simulink model "Simulacion_stepper"  (R2025b)
settings: Solver=ode4  StartTime=0.0  StopTime=Time_simulation  FixedStep=1/frecuency_simulation  RelTol=1e-3
InitFcn:
  | %%InitFcn();
StopFcn:
  | %%FinishFcn
model workspace (MAT data in the model file):
  Ts_stepper = 0.001
values from neighbouring files (symbols this model uses):
  B = motor_params.B_internal    [bode.m]    (also in current_observer.m = 0.0005; discretizacion.m = [ 1/L, 0; ekf_4_estados.m = params.B; obs_ctrl_back_emf_ext.m = [1/L 0)
  frecuency_simulation = 10e3    (= 10000)    [InitFcn.m]
  J = motor_params.J_internal    [bode.m]    (also in current_observer.m = 0.008; ekf_4_estados.m = params.J; obs_ctrl_back_emf_ext.m = 0.008; obs_y_contrl_back_emd.m = 0.008)
  Ke = 0.0055    [current_observer.m]    (also in ekf_4_estados.m = params.Ke; observer.m = Pvec(3); salient_motor.m = 0.0066)
  Ki_d = PI_dq_params.Ki_d_salient    [bode.m]
  Ki_q = PI_dq_params.Ki_q_salient    [bode.m]
  Ki_w = (wn_w^2)*J_var/Kt    [Barrido_B.m]    (also in Barrido_J.m; bode.m = PI_MTPA_params.Ki_w)
  Kp_d = PI_dq_params.Kp_d_salient    [bode.m]
  Kp_q = PI_dq_params.Kp_q_salient    [bode.m]
  Kp_w = (2*shi_w*wn_w*J_var)/Kt    [Barrido_B.m]    (also in Barrido_J.m; bode.m = PI_MTPA_params.Kp_w)
  Kt = Nr*Ke    (= 0.275)    [current_observer.m]    (also in ekf_4_estados.m = params.Kt; frecuencia_max.m = 0.33; observer.m = Pvec(4); salient_motor.m = 0.33)
  L = place(A', C', 10*eig(A)).'    [current_observer.m]    (also in desfase.m = lags(k); discretizacion.m = 0.01; frecuencia_max.m = 0.006; obs_ctrl_back_emf_ext.m = 0.006)
  P = motor_params.P    [bode.m]    (also in ekf_4_estados.m = P_pred; frecuencia_max.m = 50; salient_motor.m = 50)
  R = motor_params.R    [bode.m]    (also in current_observer.m = 3.4; discretizacion.m = 3.4; ekf_4_estados.m = params.R; frecuencia_max.m = 3.4)
  sample_time = 1/frecuency_simulation    (= 0.0001)    [InitFcn.m]
  Ts_current = 1/f_current    (= 0.0001)    [InitFcn.m]
  Ts_Wm = Ts_current*10    (= 0.001)    [InitFcn.m]
  Vdc = 24    [InitFcn.m]    (also in frecuencia_max.m = 12)
undefined symbols (not defined in the file or in its folder): DiscIntNeverNeededParam, EKF_params, motor_params, RI_base
libraries: simulink x8, mcbeeMathTransformLib x3, spspowerguiLib x1
(part 3 of 5)

== matlab function Simulacion_stepper/Motor 2 PI Speed MTPA2/MATLAB Function ==
  data: Wm_ref input; Wm input; Ts input; Kp_w input; Ki_w input; Kd_w input; Tf_w input; Tl_tdm input; B input; Imax input; RI_enable input; a_ri input; b_ri input; c_ri input; d_ri input; Kr_norm input; Ld input; Iq_ref output; Id_ref output; Iq_cogging output; Iq_PI output; Lq input; Ke input; P input; error_Wm output
function [Iq_ref, Id_ref, Iq_cogging, Iq_PI, error_Wm] = PI_speed_RI_MTPA( ...
        Wm_ref, Wm, Ts, ...
        Kp_w, Ki_w, Kd_w, Tf_w, ...
        Tl_tdm, B, ...
        Imax, ...
        RI_enable, a_ri, b_ri, c_ri, d_ri, Kr_norm, ...
        Ld, Lq, Ke, P)

% =========================================================================
% CONTROL DE VELOCIDAD Wm
%
% Incluye:
% - PI de velocidad.
% - Derivada opcional filtrada sobre la velocidad medida.
% - Compensación feedforward de carga/fricción.
% - Resonador opcional para cogging.
% - MTPA continuo.
% - Saturación vectorial de corriente.
% - Anti-windup del integrador de velocidad.
%
% Para usar solo PI:
%     Kd_w = 0;
%     RI_enable = 0;
% =========================================================================

% =========================================================================
% Estados persistentes
% =========================================================================
persistent int_w
persistent Wm_prev dWm_filt_prev
persistent y1_ri y2_ri
persistent e1_ri e2_ri

if isempty(int_w)

    int_w          = 0;

    Wm_prev        = 0;
    dWm_filt_prev  = 0;

    y1_ri          = 0;
    y2_ri          = 0;
    e1_ri          = 0;
    e2_ri          = 0;

end

% Protección numérica
Ts_eff   = max(Ts, 1e-9);
Imax_eff = max(abs(Imax), 1e-6);

% Constante de torque de reluctancia
Krel = P * (Lq - Ld);

% =========================================================================
% 1. Error de velocidad
% =========================================================================
error_Wm = Wm_ref - Wm;

% =========================================================================
% 2. Derivada filtrada sobre la velocidad medida
%
% Se usa derivada de Wm, no de error, para evitar golpes derivativos
% cuando cambia Wm_ref.
% =========================================================================
dWm_raw = (Wm - Wm_prev) / Ts_eff;

if Tf_w > 0
    alpha_d = Ts_eff / (Tf_w + Ts_eff);
    dWm_filt = dWm_filt_prev + alpha_d * (dWm_raw - dWm_filt_prev);
else
    dWm_filt = dWm_raw;
end

% Acción derivativa amortiguadora
D_w = -Kd_w * dWm_filt;

% =========================================================================
% 3. Feedforward de torque de carga y fricción
% =========================================================================
T_ff = Tl_tdm + B * Wm_ref;

if abs(Ke) > 1e-9
    Iq_ff = T_ff / Ke;
else
    Iq_ff = 0;
end

% =========================================================================
% 4. Resonador para compensación de ripple/cogging
% =========================================================================
if RI_enable == 1

    Iq_RI_new = ...
          c_ri * y1_ri ...
        - d_ri * y2_ri ...
        + Kr_norm * (error_Wm - a_ri * e1_ri + b_ri * e2_ri);

else
    Iq_RI_new = 0;
end

% =========================================================================
% 5. Integrador candidato
% =========================================================================
int_w_candidate = int_w + Ki_w * Ts_eff * error_Wm;

% =========================================================================
% 6. Cálculo PI/PID, MTPA y límite de corriente
%
% Se hacen hasta dos pasadas:
% - Primera: prueba integrando.
% - Segunda: si saturó y el integrador empeora la saturación,
%   se rechaza esa integración.
% =========================================================================
for pass = 1:2

    % Salida del controlador de velocidad
    Iq_PI = Kp_w * error_Wm + int_w_candidate + D_w;

    % Corriente q total solicitada
    Iq_ref_raw = Iq_ff + Iq_PI + Iq_RI_new;

    % =====================================================================
    % MTPA continuo
    %
    % Id_ref tiende suavemente a cero cuando Iq_ref_raw tiende a cero.
    % No existe umbral que fuerce saltos Id_ref = 0.
    % =====================================================================
    if abs(Krel) > 1e-9 && abs(Ke) > 1e-9

        A_mtpa = Ke / (2 * Krel);

        if abs(A_mtpa) > 1e-12

            % Forma numéricamente estable de:
            % Id = A - sign(A)*sqrt(A^2 + Iq^2)
            Id_ref_raw = -sign(A_mtpa) * (Iq_ref_raw^2) / ...
                (abs(A_mtpa) + sqrt(A_mtpa^2 + Iq_ref_raw^2));

        else
            Id_ref_raw = 0;
        end

    else
        Id_ref_raw = 0;
    end

    % =====================================================================
    % Saturación vectorial de corriente
    % =====================================================================
    Is_mag = sqrt(Id_ref_raw^2 + Iq_ref_raw^2);

    if Is_mag > Imax_eff

        ratio  = Imax_eff / Is_mag;

        Id_ref = Id_ref_raw * ratio;
        Iq_ref = Iq_ref_raw * ratio;

        sat = true;

    else

        Id_ref = Id_ref_raw;
        Iq_ref = Iq_ref_raw;

        sat = false;
    end

    % =====================================================================
    % Anti-windup condicional
    %
    % Si la salida está saturada y el error pide aumentar todavía más
    % la corriente saturada, no se integra.
    % Si el error ayuda a salir de saturación, sí se permite integrar.
    % =====================================================================
    integrator_worsens_sat = (Iq_ref_raw * error_Wm) >= 0;

    if pass == 1 && sat && integrator_worsens_sat

        % Rechaza la nueva integración y recalcula la salida.
        int_w_candidate = int_w;

    else
        break;
    end

end

% Guarda el integrador final
int_w = int_w_candidate;

% =========================================================================
% 7. Actualización de memorias
%
% Estas memorias se actualizan siempre, incluso durante saturación.
% =========================================================================
Wm_prev       = Wm;
dWm_filt_prev = dWm_filt;

if RI_enable == 1

    y2_ri = y1_ri;
    y1_ri = Iq_RI_new;

    e2_ri = e1_ri;
    e1_ri = error_Wm;

else

    % Evita que el resonador conserve memoria al desactivarlo.
    y1_ri = 0;
    y2_ri = 0;
    e1_ri = 0;
    e2_ri = 0;

end

% =========================================================================
% 8. Salidas de monitoreo
% =========================================================================
Iq_cogging = Iq_RI_new;

end

== matlab function Simulacion_stepper/Subsystem1/Triggered Subsystem4/MATLAB Function ==
  data: Wm_ref input; Wm input; Vd output; Vq output; Id output; Iq output; Iq_ref output; X input; Theta_e input; Ts input; Vdc input; Imax input; Kp_w input; Ki_w input; Kp_d input; Ki_d input; Kp_q input; Ki_q input; Tl_tdm input; B input; Kt input; Ke input; L input; P input; R input
function [Vd,Vq,Id,Iq,Iq_ref] = PI_dq( ...
        Wm_ref, Wm, X, Theta_e, Ts, Vdc, Imax, ...
        Kp_w, Ki_w, Kp_d, Ki_d, Kp_q, Ki_q, ...
        Tl_tdm, B, Kt, Ke, L, P,R)

% ===== FIX DIMENSIONES: preasignar salidas (escalares) =====
Vd     = 0.0;
Vq     = 0.0;
Id     = 0.0;
Iq     = 0.0;
Iq_ref = 0.0;

persistent ek_w ek1_w u_w ...
           ek_d ek1_d u_d ...
           ek_q ek1_q u_q

    if isempty(ek_w)
        ek_w  = 0;   ek1_w = 0;   u_w  = 0;
        ek_d  = 0;   ek1_d = 0;   u_d  = 0;
        ek_q  = 0;   ek1_q = 0;   u_q  = 0;
       
    end

    %% ================== Transformada dq ==================
    Ia = X(1);
    Ib = X(2);

    C = cos(Theta_e);
    S = sin(Theta_e);

    Id =  Ia*C + Ib*S;
    Iq = -Ia*S + Ib*C;   % signo correcto

    %% ================== Control de velocidad ==================
    ek1_w = ek_w;
    ek_w  = Wm_ref - Wm;

    k1_w = Kp_w + Ki_w*Ts;
    k2_w = -Kp_w;

    du_w = k1_w*ek_w + k2_w*ek1_w;
    u_w  = u_w + du_w;

    % Feedforward de torque
    Iq_ff  = (Tl_tdm + B*Wm)/Kt;
    Iq_ref = Iq_ff + u_w;

    % Saturación de corriente (Iq_ref ≤ Imax)
    if abs(Iq_ref) > Imax
        Iq_ref = sign(Iq_ref)*Imax;
        % anti-windup del PI de velocidad
        u_w  = u_w - du_w;
        ek_w = ek1_w;
    end

    %% ================== Control PI de Iq ==================
    ek1_q = ek_q;
    ek_q  = Iq_ref - Iq;

    k1_q = Kp_q + Ki_q*Ts;
    k2_q = -Kp_q;

    du_q = k1_q*ek_q + k2_q*ek1_q;
    u_q  = u_q + du_q;

    %% ================== Control PI de Id (Id_ref = 0) ==================
    ek1_d = ek_d;
    ek_d  = -Id;

    k1_d = Kp_d + Ki_d*Ts;
    k2_d = -Kp_d;

    du_d = k1_d*ek_d + k2_d*ek1_d;
    u_d  = u_d + du_d;

    %% ================== DESACOPLES ==================
    We = P * Wm;   % velocidad eléctrica

    Vdec_d = Id*R -L * We * Iq;
    Vdec_q = Iq*R + Ke * Wm + L * We * Id;

    % Voltajes no saturados
    Vd = u_d + Vdec_d;
    Vq = u_q + Vdec_q;

    %% ================== SATURACIÓN CIRCULAR dq ==================
    Vnorm = sqrt(Vd^2 + Vq^2);

    if Vnorm > Vdc
        scale = Vdc / Vnorm;
        Vd_sat = Vd * scale;
        Vq_sat = Vq * scale;

        % Anti-windup PI de corriente
        u_d = Vd_sat - Vdec_d;
        u_q = Vq_sat - Vdec_q;

        Vd = Vd_sat;
        Vq = Vq_sat;
    end

end

== matlab function Simulacion_stepper/Motor 2 PI Speed MTPA2/MATLAB Function1 ==
  data: Wm_ref input size=1; T_ref output; Wm input size=1; tl_tdm input; T_PI output; error_Wm output; Wm_filt output; PI_MTPA_params parameter
function [T_ref, T_PI, error_Wm, Wm_filt] = ...
    fcn(Wm_ref, Wm, tl_tdm, PI_MTPA_params)

[T_ref, T_PI, error_Wm, Wm_filt] = ...
    PI_speed( ...
        Wm_ref, ...
        Wm, ...
        tl_tdm, ...
        PI_MTPA_params);

end

== matlab function Simulacion_stepper/Triggered Subsystem/MATLAB Function ==
  data: Wm_cmd input; Wm_ref output; Ts input; slope input; alpha_ref output
function [Wm_ref, alpha_ref] = ramp_generator(Wm_cmd, Ts, slope)

persistent Wm_ref_prev
if isempty(Wm_ref_prev)
    Wm_ref_prev = 0;
end

delta = Wm_cmd - Wm_ref_prev;

max_step = slope * Ts;

if delta > max_step
    delta = max_step;
elseif delta < -max_step
    delta = -max_step;
end

Wm_ref = Wm_ref_prev + delta;

% 🔥 aquí está la clave
alpha_ref = (Wm_ref - Wm_ref_prev)/Ts;

Wm_ref_prev = Wm_ref;

end

== matlab function Simulacion_stepper/Subsystem1/Triggered Subsystem2/MATLAB Function ==
  data: Wm_ref input; Wm input; Vd output; Vq output; Id output; Iq output; Iq_ref output; X input; Theta_e input; Ts input; Vdc input; Imax input; Kp_w input; Ki_w input; Kp_d input; Ki_d input; Kp_q input; Ki_q input; Tl_tdm input; B input; Kt input; Ke input; L input; P input; R input
function [Vd,Vq,Id,Iq,Iq_ref] = PI_dq( ...
        Wm_ref, Wm, X, Theta_e, Ts, Vdc, Imax, ...
        Kp_w, Ki_w, Kp_d, Ki_d, Kp_q, Ki_q, ...
        Tl_tdm, B, Kt, Ke, L, P,R)

persistent ek_w ek1_w u_w ...
           ek_d ek1_d u_d ...
           ek_q ek1_q u_q

    if isempty(ek_w)
        ek_w  = 0;   ek1_w = 0;   u_w  = 0;
        ek_d  = 0;   ek1_d = 0;   u_d  = 0;
        ek_q  = 0;   ek1_q = 0;   u_q  = 0;
    end

    %% ================== Transformada dq ==================
    Ia = X(1);
    Ib = X(2);

    C = cos(Theta_e);
    S = sin(Theta_e);

    Id =  Ia*C + Ib*S;
    Iq = -Ia*S + Ib*C;   % signo correcto

    %% ================== Control de velocidad ==================
    ek1_w = ek_w;
    ek_w  = Wm_ref - Wm;

    k1_w = Kp_w + Ki_w*Ts;
    k2_w = -Kp_w;

    du_w = k1_w*ek_w + k2_w*ek1_w;
    u_w  = u_w + du_w;

    % Feedforward de torque
    Iq_ff  = (Tl_tdm + B*Wm)/Kt;
    Iq_ref = Iq_ff + u_w;

    % Saturación de corriente (Iq_ref ≤ Imax)
    if abs(Iq_ref) > Imax
        Iq_ref = sign(Iq_ref)*Imax;
        % anti-windup del PI de velocidad
        u_w  = u_w - du_w;
        ek_w = ek1_w;
    end

    %% ================== Control PI de Iq ==================
    ek1_q = ek_q;
    ek_q  = Iq_ref - Iq;

    k1_q = Kp_q + Ki_q*Ts;
    k2_q = -Kp_q;

    du_q = k1_q*ek_q + k2_q*ek1_q;
    u_q  = u_q + du_q;

    %% ================== Control PI de Id (Id_ref = 0) ==================
    ek1_d = ek_d;
    ek_d  = -Id;

    k1_d = Kp_d + Ki_d*Ts;
    k2_d = -Kp_d;

    du_d = k1_d*ek_d + k2_d*ek1_d;
    u_d  = u_d + du_d;

    %% ================== DESACOPLES ==================
    We = P * Wm;   % velocidad eléctrica

    Vdec_d = Id*R -L * We * Iq;
    Vdec_q = Iq*R + Ke * Wm + L * We * Id;

    % Voltajes no saturados
    Vd = u_d + Vdec_d;
    Vq = u_q + Vdec_q;

    %% ================== SATURACIÓN CIRCULAR dq ==================
    Vnorm = sqrt(Vd^2 + Vq^2);

    if Vnorm > Vdc
        scale = Vdc / Vnorm;
        Vd_sat = Vd * scale;
        Vq_sat = Vq * scale;

        % Anti-windup PI de corriente
        u_d = Vd_sat - Vdec_d;
        u_q = Vq_sat - Vdec_q;

        Vd = Vd_sat;
        Vq = Vq_sat;
    end

end

== matlab function Simulacion_stepper/Motor 2 PI dq/MATLAB Function ==
  data: Wm input; Vd output; X input size=[2 1]; Theta_e input; Ts input; Vdc input; Kp_d input; Ki_d input; Kp_q input; Ki_q input; Psi input; Ld input; Lq input; P input; Vq output; Id_out output; Iq_out output; Iq_ref_req input; Valpha output; Vbetha output; Amplitud_HFI input; wh input; Vd_hfi output; Vq_hfi output; HFI_enable input; Id_ref input; Iq_comp input; Kt input; error_d output; error_q output; Imax input
function [Vd, Vq, Id_out, Iq_out, ...
          Valpha, Vbetha, Vd_hfi, Vq_hfi, ...
          error_d, error_q] = PI_dq_vectorial_fixed( ...
          Wm, X, Theta_e, Ts, Vdc, ...
          Kp_d, Ki_d, Kp_q, Ki_q, ...
          Psi, Ld, Lq, P, ...
          Iq_ref_req, Amplitud_HFI, wh, HFI_enable, ...
          Id_ref, Iq_comp, Kt, Imax)

% =========================================================================
% PI dq VECTORIAL + INYECCIÓN HFI EN EJE d
%
% Salidas:
%   Vd, Vq             : tensión fundamental saturada, sin HFI
%   Vd_hfi, Vq_hfi     : tensión dq total, con HFI
%   Valpha, Vbetha     : tensión alpha-beta con HFI
%   Id_out, Iq_out     : corrientes medidas en marco dq estimado
%   error_d, error_q   : errores usados realmente por los PI
%
% Nota:
%   Imax debe representar el límite máximo del módulo de corriente:
%
%       sqrt(Id_ref^2 + Iq_ref^2) <= Imax
% =========================================================================

persistent v_int_d v_int_q
persistent t_hfi

if isempty(v_int_d)
    v_int_d = 0;
    v_int_q = 0;
    t_hfi   = 0;
end

% Protección básica
Imax = max(Imax, eps);
Ts   = max(Ts, eps);

% =========================================================================
% 1. Transformada de Park
% =========================================================================
Ia = X(1);
Ib = X(2);

cos_th = cos(Theta_e);
sin_th = sin(Theta_e);

Id =  Ia*cos_th + Ib*sin_th;
Iq = -Ia*sin_th + Ib*cos_th;

% =========================================================================
% 2. Referencia de corriente q con compensación
% =========================================================================
% La compensación se interpreta directamente como corriente equivalente.
Iq_ref_raw = Iq_ref_req - Iq_comp;

% =========================================================================
% 3. Saturación vectorial de referencias
% =========================================================================
% Primero se forma el vector solicitado completo.
I_ref_mag_raw = hypot(Id_ref, Iq_ref_raw);

if I_ref_mag_raw > Imax
    scale_I = Imax/I_ref_mag_raw;

    Id_ref_lim = Id_ref    * scale_I;
    Iq_ref_lim = Iq_ref_raw* scale_I;
else
    Id_ref_lim = Id_ref;
    Iq_ref_lim = Iq_ref_raw;
end

% =========================================================================
% 4. Errores de corriente
% =========================================================================
err_d = Id_ref_lim - Id;
err_q = Iq_ref_lim - Iq;

error_d = err_d;
error_q = err_q;

% =========================================================================
% 5. Velocidad eléctrica
% =========================================================================
We = P*Wm;

% =========================================================================
% 6. Desacople y feedforward
% =========================================================================
% Modelo:
%
%   Vd = R*Id + Ld*dId/dt - We*Lq*Iq
%   Vq = R*Iq + Lq*dIq/dt + We*Ld*Id + We*Psi
%
% Se usan las referencias limitadas en el desacople.
V_cross_d = -We*Lq*Iq_ref_lim;
V_cross_q =  We*Ld*Id_ref_lim + We*Psi;

% =========================================================================
% 7. PI sin saturar
% =========================================================================
Vd_unsat = Kp_d*err_d + v_int_d + V_cross_d;
Vq_unsat = Kp_q*err_q + v_int_q + V_cross_q;

% =========================================================================
% 8. Límite de tensión disponible
% =========================================================================
% Ajustar según el modelo del inversor:
%
%   Vdc         : si el bloque recibe directamente ese máximo vectorial.
%   Vdc/sqrt(3) : valor habitual de vector alpha-beta con SVPWM.
%
Vmax_inv = Vdc;

% Reserva conservadora para la inyección HFI.
if HFI_enable == 1
    Vmax_control = max(Vmax_inv - abs(Amplitud_HFI), 0);
else
    Vmax_control = Vmax_inv;
end

% =========================================================================
% 9. Saturación vectorial de tensión fundamental
% =========================================================================
V_mag_unsat = hypot(Vd_unsat, Vq_unsat);

if V_mag_unsat > Vmax_control && V_mag_unsat > eps
    scale_V = Vmax_control/V_mag_unsat;

    Vd = Vd_unsat*scale_V;
    Vq = Vq_unsat*scale_V;
else
    Vd = Vd_unsat;
    Vq = Vq_unsat;
end

% =========================================================================
% 10. Anti-windup por back-calculation
% =========================================================================
% Kaw tiene unidades compatibles con la ecuación del integrador.
% Este valor equivale aproximadamente a un seguimiento con constante Kp/Ki.
Kaw_d = Ki_d/max(Kp_d, eps);
Kaw_q = Ki_q/max(Kp_q, eps);

v_int_d = v_int_d + Ts*( ...
    Ki_d*err_d + Kaw_d*(Vd - Vd_unsat));

v_int_q = v_int_q + Ts*( ...
    Ki_q*err_q + Kaw_q*(Vq - Vq_unsat));

% =========================================================================
% 11. Inyección HFI
% =========================================================================
t_hfi = t_hfi + Ts;

% Evita crecimiento ilimitado del argumento temporal
if wh > 0 && t_hfi > 2*pi/wh
    t_hfi = t_hfi - 2*pi/wh;
end

if HFI_enable == 1
    v_hfi = Amplitud_HFI*sin(wh*t_hfi);
else
    v_hfi = 0;
end

% Inyección sobre el eje d estimado
Vd_hfi = Vd + v_hfi;
Vq_hfi = Vq;

% =========================================================================
% 12. Saturación final incluyendo HFI
% =========================================================================
V_mag_hfi = hypot(Vd_hfi, Vq_hfi);

if V_mag_hfi > Vmax_inv && V_mag_hfi > eps
    scale_hfi = Vmax_inv/V_mag_hfi;

    Vd_hfi = Vd_hfi*scale_hfi;
    Vq_hfi = Vq_hfi*scale_hfi;
end

% =========================================================================
% 13. Transformada inversa de Park
% =========================================================================
Valpha = Vd_hfi*cos_th - Vq_hfi*sin_th;
Vbetha = Vd_hfi*sin_th + Vq_hfi*cos_th;

% =========================================================================
% 14. Salidas de monitoreo
% =========================================================================
Id_out = Id;
Iq_out = Iq;

% Kt no se utiliza en esta versión.
% Se conserva como argumento para mantener compatibilidad con el bloque.

end

== matlab function Simulacion_stepper/Motor 2 PI Speed MTPA/MATLAB Function ==
  data: Wm_ref input; Wm input; Ts input; Kp_w input; Ki_w input; Kd_w input; Tf_w input; Tl_tdm input; B input; Imax input; RI_enable input; a_ri input; b_ri input; c_ri input; d_ri input; Kr_norm input; Ld input; Iq_ref output; Id_ref output; Iq_cogging output; Iq_PI output; Lq input; Ke input; P input; error_Wm output
function [Iq_ref, Id_ref, Iq_cogging, Iq_PI, error_Wm] = PI_speed_RI_MTPA( ...
        Wm_ref, Wm, Ts, ...
        Kp_w, Ki_w, Kd_w, Tf_w, ...
        Tl_tdm, B, ...
        Imax, ...
        RI_enable, a_ri, b_ri, c_ri, d_ri, Kr_norm, ...
        Ld, Lq, Ke, P)

% =========================================================================
% CONTROL DE VELOCIDAD Wm
%
% Incluye:
% - PI de velocidad.
% - Derivada opcional filtrada sobre la velocidad medida.
% - Compensación feedforward de carga/fricción.
% - Resonador opcional para cogging.
% - MTPA continuo.
% - Saturación vectorial de corriente.
% - Anti-windup del integrador de velocidad.
%
% Para usar solo PI:
%     Kd_w = 0;
%     RI_enable = 0;
% =========================================================================

% =========================================================================
% Estados persistentes
% =========================================================================
persistent int_w
persistent Wm_prev dWm_filt_prev
persistent y1_ri y2_ri
persistent e1_ri e2_ri

if isempty(int_w)

    int_w          = 0;

    Wm_prev        = 0;
    dWm_filt_prev  = 0;

    y1_ri          = 0;
    y2_ri          = 0;
    e1_ri          = 0;
    e2_ri          = 0;

end

% Protección numérica
Ts_eff   = max(Ts, 1e-9);
Imax_eff = max(abs(Imax), 1e-6);

% Constante de torque de reluctancia
Krel = P * (Lq - Ld);

% =========================================================================
% 1. Error de velocidad
% =========================================================================
error_Wm = Wm_ref - Wm;

% =========================================================================
% 2. Derivada filtrada sobre la velocidad medida
%
% Se usa derivada de Wm, no de error, para evitar golpes derivativos
% cuando cambia Wm_ref.
% =========================================================================
dWm_raw = (Wm - Wm_prev) / Ts_eff;

if Tf_w > 0
    alpha_d = Ts_eff / (Tf_w + Ts_eff);
    dWm_filt = dWm_filt_prev + alpha_d * (dWm_raw - dWm_filt_prev);
else
    dWm_filt = dWm_raw;
end

% Acción derivativa amortiguadora
D_w = -Kd_w * dWm_filt;

% =========================================================================
% 3. Feedforward de torque de carga y fricción
% =========================================================================
T_ff = Tl_tdm + B * Wm_ref;

if abs(Ke) > 1e-9
    Iq_ff = T_ff / Ke;
else
    Iq_ff = 0;
end

% =========================================================================
% 4. Resonador para compensación de ripple/cogging
% =========================================================================
if RI_enable == 1

    Iq_RI_new = ...
          c_ri * y1_ri ...
        - d_ri * y2_ri ...
        + Kr_norm * (error_Wm - a_ri * e1_ri + b_ri * e2_ri);

else
    Iq_RI_new = 0;
end

% =========================================================================
% 5. Integrador candidato
% =========================================================================
int_w_candidate = int_w + Ki_w * Ts_eff * error_Wm;

% =========================================================================
% 6. Cálculo PI/PID, MTPA y límite de corriente
%
% Se hacen hasta dos pasadas:
% - Primera: prueba integrando.
% - Segunda: si saturó y el integrador empeora la saturación,
%   se rechaza esa integración.
% =========================================================================
for pass = 1:2

    % Salida del controlador de velocidad
    Iq_PI = Kp_w * error_Wm + int_w_candidate + D_w;

    % Corriente q total solicitada
    Iq_ref_raw = Iq_ff + Iq_PI + Iq_RI_new;

    % =====================================================================
    % MTPA continuo
    %
    % Id_ref tiende suavemente a cero cuando Iq_ref_raw tiende a cero.
    % No existe umbral que fuerce saltos Id_ref = 0.
    % =====================================================================
    if abs(Krel) > 1e-9 && abs(Ke) > 1e-9

        A_mtpa = Ke / (2 * Krel);

        if abs(A_mtpa) > 1e-12

            % Forma numéricamente estable de:
            % Id = A - sign(A)*sqrt(A^2 + Iq^2)
            Id_ref_raw = -sign(A_mtpa) * (Iq_ref_raw^2) / ...
                (abs(A_mtpa) + sqrt(A_mtpa^2 + Iq_ref_raw^2));

        else
            Id_ref_raw = 0;
        end

    else
        Id_ref_raw = 0;
    end

    % =====================================================================
    % Saturación vectorial de corriente
    % =====================================================================
    Is_mag = sqrt(Id_ref_raw^2 + Iq_ref_raw^2);

    if Is_mag > Imax_eff

        ratio  = Imax_eff / Is_mag;

        Id_ref = Id_ref_raw * ratio;
        Iq_ref = Iq_ref_raw * ratio;

        sat = true;

    else

        Id_ref = Id_ref_raw;
        Iq_ref = Iq_ref_raw;

        sat = false;
    end

    % =====================================================================
    % Anti-windup condicional
    %
    % Si la salida está saturada y el error pide aumentar todavía más
    % la corriente saturada, no se integra.
    % Si el error ayuda a salir de saturación, sí se permite integrar.
    % =====================================================================
    integrator_worsens_sat = (Iq_ref_raw * error_Wm) >= 0;

    if pass == 1 && sat && integrator_worsens_sat

        % Rechaza la nueva integración y recalcula la salida.
        int_w_candidate = int_w;

    else
        break;
    end

end

% Guarda el integrador final
int_w = int_w_candidate;

% =========================================================================
% 7. Actualización de memorias
%
% Estas memorias se actualizan siempre, incluso durante saturación.
% =========================================================================
Wm_prev       = Wm;
dWm_filt_prev = dWm_filt;

if RI_enable == 1

    y2_ri = y1_ri;
    y1_ri = Iq_RI_new;

    e2_ri = e1_ri;
    e1_ri = error_Wm;

else

    % Evita que el resonador conserve memoria al desactivarlo.
    y1_ri = 0;
    y2_ri = 0;
    e1_ri = 0;
    e2_ri = 0;

end

% =========================================================================
% 8. Salidas de monitoreo
% =========================================================================
Iq_cogging = Iq_RI_new;

end

== matlab function Simulacion_stepper/Motor 1  Speed PR/MATLAB Function ==
  data: Wm_ref input; Wm input; Ts input; Kp_w input; Ki_w input; Kd_w input; Tf_w input; Tl_tdm input; B input; Imax input; RI_enable input; a_ri input; b_ri input; c_ri input; d_ri input; Kr_norm input; Ld input; Iq_ref output; Id_ref output; Iq_cogging output; Iq_PI output; Lq input; Ke input; P input; error_Wm output
function [Iq_ref, Id_ref, Iq_cogging, Iq_PI, error_Wm] = PI_speed_RI_MTPA( ...
        Wm_ref, Wm, Ts, ...
        Kp_w, Ki_w, Kd_w, Tf_w, ...
        Tl_tdm, B, ...
        Imax, ...
        RI_enable, a_ri, b_ri, c_ri, d_ri, Kr_norm, ...
        Ld, Lq, Ke, P)

% =========================================================================
% CONTROL DE VELOCIDAD Wm
%
% Incluye:
% - PI de velocidad.
% - Derivada opcional filtrada sobre la velocidad medida.
% - Compensación feedforward de carga/fricción.
% - Resonador opcional para cogging.
% - MTPA continuo.
% - Saturación vectorial de corriente.
% - Anti-windup del integrador de velocidad.
%
% Para usar solo PI:
%     Kd_w = 0;
%     RI_enable = 0;
% =========================================================================

% =========================================================================
% Estados persistentes
% =========================================================================
persistent int_w
persistent Wm_prev dWm_filt_prev
persistent y1_ri y2_ri
persistent e1_ri e2_ri

if isempty(int_w)

    int_w          = 0;

    Wm_prev        = 0;
    dWm_filt_prev  = 0;

    y1_ri          = 0;
    y2_ri          = 0;
    e1_ri          = 0;
    e2_ri          = 0;

end

% Protección numérica
Ts_eff   = max(Ts, 1e-9);
Imax_eff = max(abs(Imax), 1e-6);

% Constante de torque de reluctancia
Krel = P * (Lq - Ld);

% =========================================================================
% 1. Error de velocidad
% =========================================================================
error_Wm = Wm_ref - Wm;

% =========================================================================
% 2. Derivada filtrada sobre la velocidad medida
%
% Se usa derivada de Wm, no de error, para evitar golpes derivativos
% cuando cambia Wm_ref.
% =========================================================================
dWm_raw = (Wm - Wm_prev) / Ts_eff;

if Tf_w > 0
    alpha_d = Ts_eff / (Tf_w + Ts_eff);
    dWm_filt = dWm_filt_prev + alpha_d * (dWm_raw - dWm_filt_prev);
else
    dWm_filt = dWm_raw;
end

% Acción derivativa amortiguadora
D_w = -Kd_w * dWm_filt;

% =========================================================================
% 3. Feedforward de torque de carga y fricción
% =========================================================================
T_ff = Tl_tdm + B * Wm_ref;

if abs(Ke) > 1e-9
    Iq_ff = T_ff / Ke;
else
    Iq_ff = 0;
end

% =========================================================================
% 4. Resonador para compensación de ripple/cogging
% =========================================================================
if RI_enable == 1

    Iq_RI_new = ...
          c_ri * y1_ri ...
        - d_ri * y2_ri ...
        + Kr_norm * (error_Wm - a_ri * e1_ri + b_ri * e2_ri);

else
    Iq_RI_new = 0;
end

% =========================================================================
% 5. Integrador candidato
% =========================================================================
int_w_candidate = int_w + Ki_w * Ts_eff * error_Wm;

% =========================================================================
% 6. Cálculo PI/PID, MTPA y límite de corriente
%
% Se hacen hasta dos pasadas:
% - Primera: prueba integrando.
% - Segunda: si saturó y el integrador empeora la saturación,
%   se rechaza esa integración.
% =========================================================================
for pass = 1:2

    % Salida del controlador de velocidad
    Iq_PI = Kp_w * error_Wm + int_w_candidate + D_w;

    % Corriente q total solicitada
    Iq_ref_raw = Iq_ff + Iq_PI + Iq_RI_new;

    % =====================================================================
    % MTPA continuo
    %
    % Id_ref tiende suavemente a cero cuando Iq_ref_raw tiende a cero.
    % No existe umbral que fuerce saltos Id_ref = 0.
    % =====================================================================
    if abs(Krel) > 1e-9 && abs(Ke) > 1e-9

        A_mtpa = Ke / (2 * Krel);

        if abs(A_mtpa) > 1e-12

            % Forma numéricamente estable de:
            % Id = A - sign(A)*sqrt(A^2 + Iq^2)
            Id_ref_raw = -sign(A_mtpa) * (Iq_ref_raw^2) / ...
                (abs(A_mtpa) + sqrt(A_mtpa^2 + Iq_ref_raw^2));

        else
            Id_ref_raw = 0;
        end

    else
        Id_ref_raw = 0;
    end

    % =====================================================================
    % Saturación vectorial de corriente
    % =====================================================================
    Is_mag = sqrt(Id_ref_raw^2 + Iq_ref_raw^2);

    if Is_mag > Imax_eff

        ratio  = Imax_eff / Is_mag;

        Id_ref = Id_ref_raw * ratio;
        Iq_ref = Iq_ref_raw * ratio;

        sat = true;

    else

        Id_ref = Id_ref_raw;
        Iq_ref = Iq_ref_raw;

        sat = false;
    end

    % =====================================================================
    % Anti-windup condicional
    %
    % Si la salida está saturada y el error pide aumentar todavía más
    % la corriente saturada, no se integra.
    % Si el error ayuda a salir de saturación, sí se permite integrar.
    % =====================================================================
    integrator_worsens_sat = (Iq_ref_raw * error_Wm) >= 0;

    if pass == 1 && sat && integrator_worsens_sat

        % Rechaza la nueva integración y recalcula la salida.
        int_w_candidate = int_w;

    else
        break;
    end

end

% Guarda el integrador final
int_w = int_w_candidate;

% =========================================================================
% 7. Actualización de memorias
%
% Estas memorias se actualizan siempre, incluso durante saturación.
% =========================================================================
Wm_prev       = Wm;
dWm_filt_prev = dWm_filt;

if RI_enable == 1

    y2_ri = y1_ri;
    y1_ri = Iq_RI_new;

    e2_ri = e1_ri;
    e1_ri = error_Wm;

else

    % Evita que el resonador conserve memoria al desactivarlo.
    y1_ri = 0;
    y2_ri = 0;
    e1_ri = 0;
    e2_ri = 0;

end

% =========================================================================
% 8. Salidas de monitoreo
% =========================================================================
Iq_cogging = Iq_RI_new;

end

== matlab function Simulacion_stepper/Motor 1  Speed PR/MATLAB Function1 ==
  data: Wm_ref input size=1; Vq_res output; Wm input size=1; error_res output; RI_params_M1 parameter; V_inphase output; V_quadrature output
function [Vq_res, error_res, V_inphase, V_quadrature] = ...
    fcn(Wm_ref, Wm, RI_params_M1)

[Vq_res, error_res, V_inphase, V_quadrature] = ...
    resonant_speed( ...
        Wm_ref, Wm, RI_params_M1);

end

== matlab function Simulacion_stepper/Motor 2 PI dq1/MATLAB Function ==
  data: Wm input; Vd output; X input size=[2 1]; Theta_e input; Ts input; Vdc input; Kp_d input; Ki_d input; Kp_q input; Ki_q input; Psi input; Ld input; Lq input; P input; Vq output; Id_out output; Iq_out output; Iq_ref_req input; Valpha output; Vbetha output; Amplitud_HFI input; wh input; Vd_hfi output; Vq_hfi output; HFI_enable input; Id_ref input; Iq_comp input; Kt input; error_d output; error_q output; Imax input
function [Vd, Vq, Id_out, Iq_out, ...
          Valpha, Vbetha, Vd_hfi, Vq_hfi, ...
          error_d, error_q] = PI_dq_vectorial_fixed( ...
          Wm, X, Theta_e, Ts, Vdc, ...
          Kp_d, Ki_d, Kp_q, Ki_q, ...
          Psi, Ld, Lq, P, ...
          Iq_ref_req, Amplitud_HFI, wh, HFI_enable, ...
          Id_ref, Iq_comp, Kt, Imax)

% =========================================================================
% PI dq VECTORIAL + INYECCIÓN HFI EN EJE d
%
% Salidas:
%   Vd, Vq             : tensión fundamental saturada, sin HFI
%   Vd_hfi, Vq_hfi     : tensión dq total, con HFI
%   Valpha, Vbetha     : tensión alpha-beta con HFI
%   Id_out, Iq_out     : corrientes medidas en marco dq estimado
%   error_d, error_q   : errores usados realmente por los PI
%
% Nota:
%   Imax debe representar el límite máximo del módulo de corriente:
%
%       sqrt(Id_ref^2 + Iq_ref^2) <= Imax
% =========================================================================

persistent v_int_d v_int_q
persistent t_hfi

if isempty(v_int_d)
    v_int_d = 0;
    v_int_q = 0;
    t_hfi   = 0;
end

% Protección básica
Imax = max(Imax, eps);
Ts   = max(Ts, eps);

% =========================================================================
% 1. Transformada de Park
% =========================================================================
Ia = X(1);
Ib = X(2);

cos_th = cos(Theta_e);
sin_th = sin(Theta_e);

Id =  Ia*cos_th + Ib*sin_th;
Iq = -Ia*sin_th + Ib*cos_th;

% =========================================================================
% 2. Referencia de corriente q con compensación
% =========================================================================
% La compensación se interpreta directamente como corriente equivalente.
Iq_ref_raw = Iq_ref_req - Iq_comp;

% =========================================================================
% 3. Saturación vectorial de referencias
% =========================================================================
% Primero se forma el vector solicitado completo.
I_ref_mag_raw = hypot(Id_ref, Iq_ref_raw);

if I_ref_mag_raw > Imax
    scale_I = Imax/I_ref_mag_raw;

    Id_ref_lim = Id_ref    * scale_I;
    Iq_ref_lim = Iq_ref_raw* scale_I;
else
    Id_ref_lim = Id_ref;
    Iq_ref_lim = Iq_ref_raw;
end

% =========================================================================
% 4. Errores de corriente
% =========================================================================
err_d = Id_ref_lim - Id;
err_q = Iq_ref_lim - Iq;

error_d = err_d;
error_q = err_q;

% =========================================================================
% 5. Velocidad eléctrica
% =========================================================================
We = P*Wm;

% =========================================================================
% 6. Desacople y feedforward
% =========================================================================
% Modelo:
%
%   Vd = R*Id + Ld*dId/dt - We*Lq*Iq
%   Vq = R*Iq + Lq*dIq/dt + We*Ld*Id + We*Psi
%
% Se usan las referencias limitadas en el desacople.
V_cross_d = -We*Lq*Iq_ref_lim;
V_cross_q =  We*Ld*Id_ref_lim + We*Psi;

% =========================================================================
% 7. PI sin saturar
% =========================================================================
Vd_unsat = Kp_d*err_d + v_int_d + V_cross_d;
Vq_unsat = Kp_q*err_q + v_int_q + V_cross_q;

% =========================================================================
% 8. Límite de tensión disponible
% =========================================================================
% Ajustar según el modelo del inversor:
%
%   Vdc         : si el bloque recibe directamente ese máximo vectorial.
%   Vdc/sqrt(3) : valor habitual de vector alpha-beta con SVPWM.
%
Vmax_inv = Vdc;

% Reserva conservadora para la inyección HFI.
if HFI_enable == 1
    Vmax_control = max(Vmax_inv - abs(Amplitud_HFI), 0);
else
    Vmax_control = Vmax_inv;
end

% =========================================================================
% 9. Saturación vectorial de tensión fundamental
% =========================================================================
V_mag_unsat = hypot(Vd_unsat, Vq_unsat);

if V_mag_unsat > Vmax_control && V_mag_unsat > eps
    scale_V = Vmax_control/V_mag_unsat;

    Vd = Vd_unsat*scale_V;
    Vq = Vq_unsat*scale_V;
else
    Vd = Vd_unsat;
    Vq = Vq_unsat;
end

% =========================================================================
% 10. Anti-windup por back-calculation
% =========================================================================
% Kaw tiene unidades compatibles con la ecuación del integrador.
% Este valor equivale aproximadamente a un seguimiento con constante Kp/Ki.
Kaw_d = Ki_d/max(Kp_d, eps);
Kaw_q = Ki_q/max(Kp_q, eps);

v_int_d = v_int_d + Ts*( ...
    Ki_d*err_d + Kaw_d*(Vd - Vd_unsat));

v_int_q = v_int_q + Ts*( ...
    Ki_q*err_q + Kaw_q*(Vq - Vq_unsat));

% =========================================================================
% 11. Inyección HFI
% =========================================================================
t_hfi = t_hfi + Ts;

% Evita crecimiento ilimitado del argumento temporal
if wh > 0 && t_hfi > 2*pi/wh
    t_hfi = t_hfi - 2*pi/wh;
end

if HFI_enable == 1
    v_hfi = Amplitud_HFI*sin(wh*t_hfi);
else
    v_hfi = 0;
end

% Inyección sobre el eje d estimado
Vd_hfi = Vd + v_hfi;
Vq_hfi = Vq;

% =========================================================================
% 12. Saturación final incluyendo HFI
% =========================================================================
V_mag_hfi = hypot(Vd_hfi, Vq_hfi);

if V_mag_hfi > Vmax_inv && V_mag_hfi > eps
    scale_hfi = Vmax_inv/V_mag_hfi;

    Vd_hfi = Vd_hfi*scale_hfi;
    Vq_hfi = Vq_hfi*scale_hfi;
end

% =========================================================================
% 13. Transformada inversa de Park
% =========================================================================
Valpha = Vd_hfi*cos_th - Vq_hfi*sin_th;
Vbetha = Vd_hfi*sin_th + Vq_hfi*cos_th;

% =========================================================================
% 14. Salidas de monitoreo
% =========================================================================
Id_out = Id;
Iq_out = Iq;

% Kt no se utiliza en esta versión.
% Se conserva como argumento para mantener compatibilidad con el bloque.

end

== matlab function Simulacion_stepper/Motor 2 PI dq1/MATLAB Function1 ==
  data: Wm input; Vd output; X input; Theta_e input; T_ref input; comp_res input; Vq output; Id_out output; Iq_out output; Valpha output; Vbetha output; Vd_hfi output; Vq_hfi output; error_d output; error_q output; PI_dq_params parameter; Id_ref_out output; Iq_ref_out output; T_ref_real output
function [Vd, Vq, Id_out, Iq_out, ...
          Valpha, Vbetha, Vd_hfi, Vq_hfi, ...
          error_d, error_q, ...
          Id_ref_out, Iq_ref_out, T_ref_real] = ...
    fcn(Wm, X, Theta_e, T_ref,comp_res, PI_dq_params)

[Vd, Vq, Id_out, Iq_out, ...
          Valpha, Vbetha, Vd_hfi, Vq_hfi, ...
          error_d, error_q, ...
          Id_ref_out, Iq_ref_out, T_ref_real] = ...
    PI_dq( ...
        Wm, ...
        X, ...
        Theta_e, ...
        T_ref,...
        comp_res,...
        PI_dq_params);

end
